simulink model "simrfV2_TX_array"  (R2022b)
settings: Solver=FixedStepDiscrete  StartTime=0.0  StopTime=15e-8  RelTol=1e-3
PreLoadFcn:
  | % Init values just to make sure that the model is loaded correctly when
  | % not run within example script:
  | if ~exist('arrayTXObj','var')
  |     % General properties:
  |     TX_Pin = -7.41; % Transmitter input power (dBm)
  |     CF = 35e9; % Center frequency (Hz)
  |     lambda = physconst('lightspeed')/CF; % Wavelength (1/m)
  |     d = 100*lambda; % Distance between TX and RX antennas (m)
  |     DOD = 180; % Direction of departure (deg)
  |     % Antenna properties:
  |     arrayTXObj = design(linearArray, CF, dipole);
  |     arrayTXObj.NumElements = 8;
  |     arrayTXObj.TiltAxis = [0 0 1];
  |     arrayTXObj.Tilt = 180;
  |     % antenna S-parameters - antenna should be pre-solved before used in block
  |     sp = sparameters(arrayTXObj,CF);
  |     Az_TX = 90-DOD; % Azimuth Direction of departure
  |     El_TX = 0; % Elevation of Direction of departure
  |     % RF system Properties:
  |     Beam_Az_TX = DOD; % Beamforming angle (deg)
  |     beamformer = phased.PhaseShiftBeamformer(...
  |         'SensorArray',phased.ULA('NumElements',8,...
  |         'ElementSpacing', lambda/2), ...
  |         'OperatingFrequency',CF,...
  |         'Direction',[Beam_Az_TX; 0],...
  |         'WeightsOutputPort',true);
  |     [~, phase_shifts_TX] = beamformer(ones(1,8));
  |     phase_shifts_TX = angle(phase_shifts_TX)'/pi*180;
  |     G_TX = 18.6*ones(1,8); % Added gain of each RF chain
  |     oIP3_TX = 30; % 3rd order output intercept point (dBm)
  | end
values from neighbouring files (symbols this model uses):
  Bias = 0    [ModelingRFSystemsWithAntennaArraysUsingAntennaBlockExample.m]    (also in beam_control_ic_rx_parameter.m)
  fbb = ones(8)    [ModelingRFSystemsWithAntennaArraysUsingAntennaBlockExample.m]
libraries: dspfdesign x1, dspsigops x1
settings Model: SimulationMode=accelerator  Creator=The MathWorks, Inc.  LastModifiedBy=User
settings SolverCC: AlgebraicLoopSolver=TrustRegion  MaxZcPerStep=1
settings DataIOCC: SaveOutput=off  SignalLogging=off  DSMLogging=off  SaveTime=off  ReturnWorkspaceOutputs=off
settings DebuggingCC: InheritedTsInSrcMsg=none  UnconnectedInputMsg=warning  UnconnectedOutputMsg=warning  UnconnectedLineMsg=warning  SFMachineParentedDataDiag=warning
settings ModelReferenceCC: EnableRefExpFcnMdlSchedulingChecks=on
settings RTWCC: DLArmComputeVersion=19.05

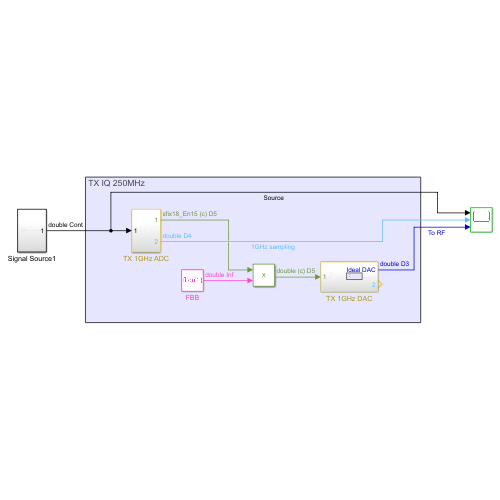
[thumbnail: Simulink's stored preview of the top-level diagram]
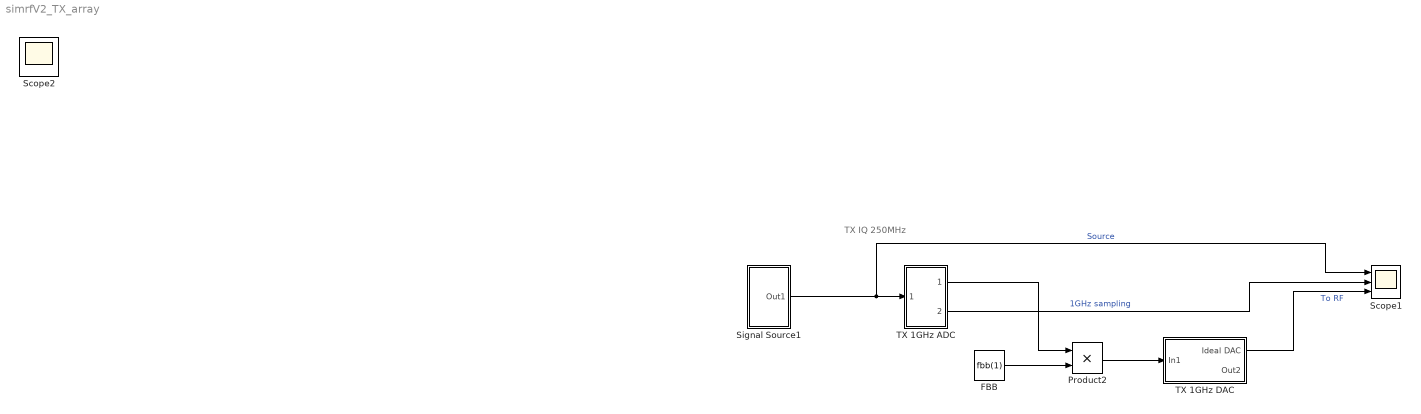
== system simrfV2_TX_array ==
  note: TX IQ 250MHz
  FBB : Constant  Value=fbb(1)
  Product2 : Product
  Scope1 : Scope  NumInputPorts=3
  Signal Source1 : Subsystem
  TX 1GHz ADC : Subsystem
  TX 1GHz DAC : Subsystem
  Scope2 : Scope
  wires:
  TX 1GHz DAC/1(Ideal DAC) -> Scope1/3  "To RF"
  TX 1GHz ADC/2(Out2) -> Scope1/2  "1GHz sampling"
  TX 1GHz ADC/1(Out1) -> Product2/1
  Signal Source1/1(Out1) -> TX 1GHz ADC/1(In1), Scope1/1  "Source"
  FBB/1 -> Product2/2
  Product2/1 -> TX 1GHz DAC/1(In1)

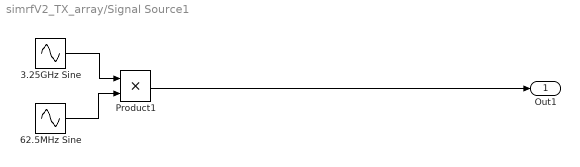
== system simrfV2_TX_array/Signal Source1 ==
  3.25GHz Sine : Sin  Frequency=2*pi*3.25e9  SampleTime=0
  62.5MHz Sine : Sin  Frequency=2*pi*62.5e6  SampleTime=0
  Product1 : Product
  Out1 : Outport
  wires:
  3.25GHz Sine/1 -> Product1/1
  62.5MHz Sine/1 -> Product1/2
  Product1/1 -> Out1/1

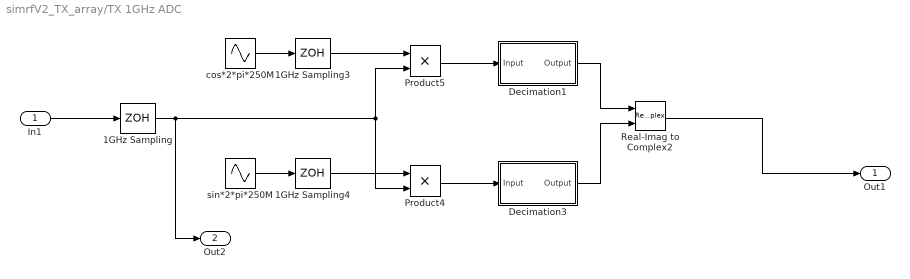
== system simrfV2_TX_array/TX 1GHz ADC ==
  In1 : Inport
  1GHz Sampling : ZeroOrderHold  SampleTime=1/1e9
  1GHz Sampling3 : ZeroOrderHold  SampleTime=1/1e9
  1GHz Sampling4 : ZeroOrderHold  SampleTime=1/1e9
  Decimation1 : Subsystem  Tag=FilterWizardSubSystem
      settings: ErrorFcn=dspFilterRealizedInBasicElemsAlgLoopErrFcnCallback
  Decimation3 : Subsystem  Tag=FilterWizardSubSystem
      settings: ErrorFcn=dspFilterRealizedInBasicElemsAlgLoopErrFcnCallback
  Product4 : Product
  Product5 : Product
  Real-Imag to Complex2 : RealImagToComplex
  cos*2*pi*250M : Sin  Frequency=2*pi*250e6  Phase=1.5707  SampleTime=0
  sin*2*pi*250M : Sin  Frequency=2*pi*250e6  SampleTime=0
  Out1 : Outport
  Out2 : Outport  Port=2
  wires:
  Product4/1 -> Decimation3/1(Input)
  Decimation1/1(Output) -> Real-Imag to Complex2/1
  sin*2*pi*250M/1 -> 1GHz Sampling4/1
  1GHz Sampling4/1 -> Product4/1
  1GHz Sampling3/1 -> Product5/1
  Product5/1 -> Decimation1/1(Input)
  1GHz Sampling/1 -> Out2/1, Product4/2, Product5/2
  cos*2*pi*250M/1 -> 1GHz Sampling3/1
  Decimation3/1(Output) -> Real-Imag to Complex2/2
  In1/1 -> 1GHz Sampling/1
  Real-Imag to Complex2/1 -> Out1/1

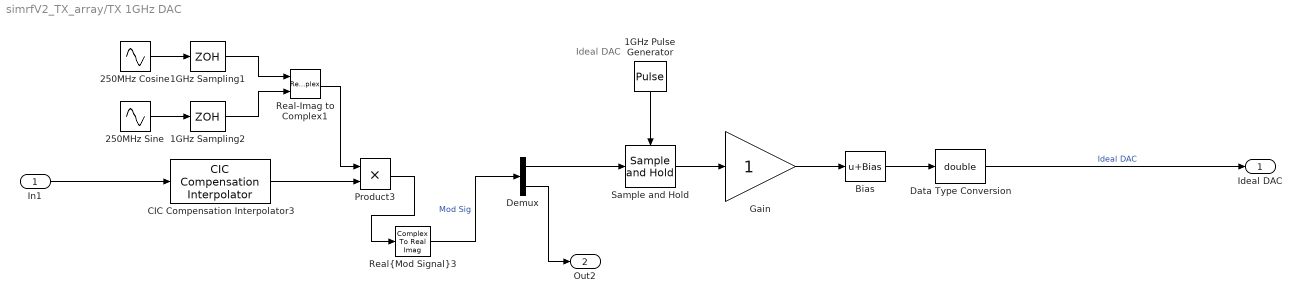
== system simrfV2_TX_array/TX 1GHz DAC ==
  note: Ideal DAC
  In1 : Inport
  1GHz Pulse Generator : DiscretePulseGenerator  PulseType=Time based  Period=1 / 1e9  PulseWidth=50
  1GHz Sampling1 : ZeroOrderHold  SampleTime=1/1e9
  1GHz Sampling2 : ZeroOrderHold  SampleTime=1/1e9
  250MHz Cosine : Sin  Frequency=2*pi*250e6  Phase=1.5707  SampleTime=0
  250MHz Sine : Sin  Frequency=2*pi*250e6  SampleTime=0
  Bias : Bias  Bias=Bias  SaturateOnIntegerOverflow=off
  CIC Compensation Interpolator3 : dspfdesign/CIC Compensation Interpolator  CICRateChangeFactor=2  CICNumSections=4  CICDifferentialDelay=1  InterpolationFactor=2  DesignForMinimumOrder=on  FilterOrder=12  PassbandFrequency=2.5e8  StopbandFrequency=3.25e8  PassbandRipple=0.1  StopbandAttenuation=60  InheritSampleRate=off  SampleRate=1e9  SimulateUsing=Interpreted execution  roundingMode=Floor  coeffsDataTypeStr=fixdt(1,16)
  Data Type Conversion : DataTypeConversion  OutDataTypeStr=double  SaturateOnIntegerOverflow=off  RndMeth=Floor
  Demux : Demux  Outputs=2
  Gain : Gain
  Product3 : Product
  Real-Imag to Complex1 : RealImagToComplex
  "Real{Mod Signal}3" : ComplexToRealImag  Output=Real
  Sample and Hold : dspsigops/Sample and Hold  trig=Rising edge  initCond=0  latchinput=off
  Ideal DAC : Outport
  Out2 : Outport  Port=2
  wires:
  Gain/1 -> Bias/1
  1GHz Sampling2/1 -> Real-Imag to Complex1/2
  CIC Compensation Interpolator3/1 -> Product3/2
  1GHz Pulse Generator/1 -> Sample and Hold/Trigger
  1GHz Sampling1/1 -> Real-Imag to Complex1/1
  Real-Imag to Complex1/1 -> Product3/1
  Product3/1 -> "Real{Mod Signal}3"/1
  250MHz Sine/1 -> 1GHz Sampling2/1
  "Real{Mod Signal}3"/1 -> Demux/1  "Mod Sig"
  250MHz Cosine/1 -> 1GHz Sampling1/1
  Bias/1 -> Data Type Conversion/1
  Sample and Hold/1 -> Gain/1
  Demux/2 -> Out2/1
  Demux/1 -> Sample and Hold/1
  In1/1 -> CIC Compensation Interpolator3/1
  Data Type Conversion/1 -> Ideal DAC/1  "Ideal DAC"

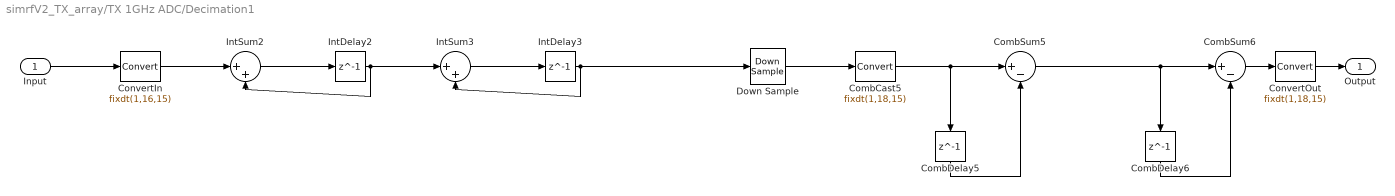
== system simrfV2_TX_array/TX 1GHz ADC/Decimation1 ==
  Input : Inport
  CombCast5 : DataTypeConversion  OutDataTypeStr=fixdt(1,18,15)  SaturateOnIntegerOverflow=off  RndMeth=Floor
  CombDelay5 : Delay  DelayLength=1  InitialCondition=0
  CombDelay6 : Delay  DelayLength=1  InitialCondition=0
  CombSum5 : Sum  Inputs=|+-  AccumDataTypeStr=fixdt(1,18,15)  OutDataTypeStr=fixdt(1,18,15)
  CombSum6 : Sum  Inputs=|+-  AccumDataTypeStr=fixdt(1,18,15)  OutDataTypeStr=fixdt(1,18,15)
  ConvertIn : DataTypeConversion  OutDataTypeStr=fixdt(1,16,15)  RndMeth=Nearest
  ConvertOut : DataTypeConversion  OutDataTypeStr=fixdt(1,18,15)  SaturateOnIntegerOverflow=off  RndMeth=Floor
  Down Sample : DownSample  RateOptions=Allow multirate processing  AllowArbitraryFixedInput=on
  IntDelay2 : Delay  DelayLength=1  InitialCondition=0
  IntDelay3 : Delay  DelayLength=1  InitialCondition=0
  IntSum2 : Sum  Inputs=|++  AccumDataTypeStr=fixdt(1,18,15)  OutDataTypeStr=fixdt(1,18,15)
  IntSum3 : Sum  Inputs=|++  AccumDataTypeStr=fixdt(1,18,15)  OutDataTypeStr=fixdt(1,18,15)
  Output : Outport
  wires:
  Input/1 -> ConvertIn/1
  ConvertIn/1 -> IntSum2/1
  IntSum2/1 -> IntDelay2/1
  IntDelay2/1 -> IntSum2/2, IntSum3/1
  IntSum3/1 -> IntDelay3/1
  IntDelay3/1 -> IntSum3/2, Down Sample/1
  Down Sample/1 -> CombCast5/1
  CombSum5/1 -> CombSum6/1, CombDelay6/1
  CombDelay5/1 -> CombSum5/2
  CombCast5/1 -> CombSum5/1, CombDelay5/1
  CombSum6/1 -> ConvertOut/1
  CombDelay6/1 -> CombSum6/2
  ConvertOut/1 -> Output/1

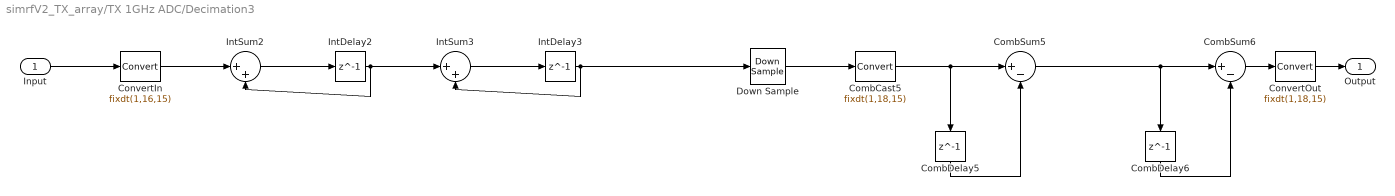
== system simrfV2_TX_array/TX 1GHz ADC/Decimation3 ==
  Input : Inport
  CombCast5 : DataTypeConversion  OutDataTypeStr=fixdt(1,18,15)  SaturateOnIntegerOverflow=off  RndMeth=Floor
  CombDelay5 : Delay  DelayLength=1  InitialCondition=0
  CombDelay6 : Delay  DelayLength=1  InitialCondition=0
  CombSum5 : Sum  Inputs=|+-  AccumDataTypeStr=fixdt(1,18,15)  OutDataTypeStr=fixdt(1,18,15)
  CombSum6 : Sum  Inputs=|+-  AccumDataTypeStr=fixdt(1,18,15)  OutDataTypeStr=fixdt(1,18,15)
  ConvertIn : DataTypeConversion  OutDataTypeStr=fixdt(1,16,15)  RndMeth=Nearest
  ConvertOut : DataTypeConversion  OutDataTypeStr=fixdt(1,18,15)  SaturateOnIntegerOverflow=off  RndMeth=Floor
  Down Sample : DownSample  RateOptions=Allow multirate processing  AllowArbitraryFixedInput=on
  IntDelay2 : Delay  DelayLength=1  InitialCondition=0
  IntDelay3 : Delay  DelayLength=1  InitialCondition=0
  IntSum2 : Sum  Inputs=|++  AccumDataTypeStr=fixdt(1,18,15)  OutDataTypeStr=fixdt(1,18,15)
  IntSum3 : Sum  Inputs=|++  AccumDataTypeStr=fixdt(1,18,15)  OutDataTypeStr=fixdt(1,18,15)
  Output : Outport
  wires:
  ConvertOut/1 -> Output/1
  CombDelay6/1 -> CombSum6/2
  CombSum6/1 -> ConvertOut/1
  CombCast5/1 -> CombDelay5/1, CombSum5/1
  CombDelay5/1 -> CombSum5/2
  CombSum5/1 -> CombDelay6/1, CombSum6/1
  Down Sample/1 -> CombCast5/1
  IntDelay3/1 -> Down Sample/1, IntSum3/2
  IntSum3/1 -> IntDelay3/1
  IntDelay2/1 -> IntSum3/1, IntSum2/2
  IntSum2/1 -> IntDelay2/1
  ConvertIn/1 -> IntSum2/1
  Input/1 -> ConvertIn/1
